simulink model "PID_AW_c"  (R2015b)
settings: Solver=VariableStepAuto  StartTime=0.0  StopTime=10.0  RelTol=1e-3
undefined symbols (not defined in the file): D, I, N, P, sat_lim_max, sat_lim_min
settings Model: Creator=mgreiff  LastModifiedBy=mgreiff

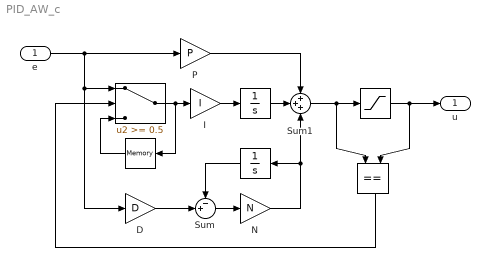
== system PID_AW_c ==
  e : Inport
  " " : Integrator
  "  " : Saturate  UpperLimit=sat_lim_max  LowerLimit=sat_lim_min
  "   " : Integrator
  "    " : Memory
  "     " : Switch  Threshold=0.5
  "       " : RelationalOperator  Operator===  OutDataTypeStr=boolean
  D : Gain  Gain=D
  I : Gain  Gain=I
  N : Gain  Gain=N
  P : Gain  Gain=P
  Sum : Sum  Inputs=-+|
  Sum1 : Sum  Inputs=+++
  u : Outport
  wires:
  e/1 -> D/1, "     "/1, P/1
  D/1 -> Sum/2
  Sum/1 -> N/1
  I/1 -> " "/1
  N/1 -> "   "/1, Sum1/3
  "   "/1 -> Sum/1
  P/1 -> Sum1/1
  " "/1 -> Sum1/2
  "    "/1 -> "     "/3
  "       "/1 -> "     "/2
  "     "/1 -> "    "/1, I/1
  Sum1/1 -> "  "/1, "       "/1
  "  "/1 -> "       "/2, u/1
